simulink model "SIMULACION"  (R2025a)
settings: Solver=VariableStepAuto  StartTime=0.0  StopTime=100  RelTol=1e-3
values from neighbouring files (symbols this model uses):
  A = [0 1 0; -2.9856 -0.2654 0; -0.2985 0 0]    [Ackerman.m]    (also in L1.m = [0 1 0 0; Lab1.m = [0 1 0 0)
  Ac_poly = [0 1 0 0 ... (first row only)    [L1.m]    (also in Lab1.m)
  amp = 1    [L1.m]
  Ao_poly = [0 0 0 -den(5) ... (first row only)    [L1.m]    (also in Lab1.m)
  Ap = Ac_poly    [L1.m]    (also in Lab1.m = A)
  B = [0; 1; 0]    [Ackerman.m]    (also in L1.m = [0; 1/m; 0; -1/(m*L)]; Lab1.m = [0; 1/m; 0; -1/(m*L)])
  Bc_poly = [0; 0; 0; 1]    [L1.m]    (also in Lab1.m)
  Bo_poly = [num(5)-(den(5)*num(1)) ... (first row only)    [L1.m]    (also in Lab1.m)
  Bp = Bc_poly    [L1.m]    (also in Lab1.m = B)
  C = [1 0 0 0]    [L1.m]    (also in Lab1.m)
  Cc_poly = [num(5)-(den(5)*num(1))  num(4)-(den(4)*num(1))             num(3)-(den(3)*num(1))  num(2)-(den(2)*num(1))]    [L1.m]    (also in Lab1.m)
  Co_poly = [0 0 0 1]    [L1.m]    (also in Lab1.m)
  Cp = Cc_poly    [L1.m]    (also in Lab1.m = C)
  E = [0; M/m; 0; -M + m/L*m]    [L1.m]    (also in Lab1.m)
  sol_ki = double(sol.ki)    [L1.m]    (also in Lab1.m)
  sol_vector = double(k_valores)    [L1.m]    (also in Lab1.m)
  w = 1    [L1.m]

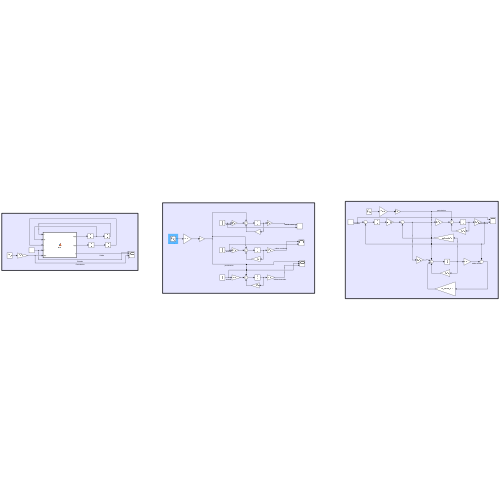
[thumbnail: Simulink's stored preview of the top-level diagram]
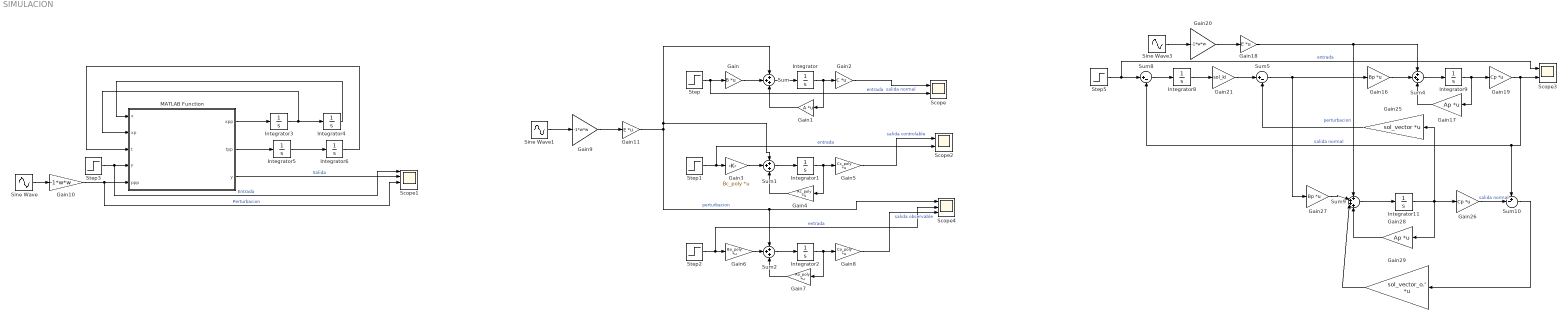
== system SIMULACION ==
  Gain : Gain  Gain=B  Multiplication=Matrix(K*u)
  Gain1 : Gain  Gain=A  Multiplication=Matrix(K*u)
  Gain10 : Gain  Gain=-1*w*w
  Gain11 : Gain  Gain=E  Multiplication=Matrix(K*u)
  Gain16 : Gain  Gain=Bp  Multiplication=Matrix(K*u)
  Gain17 : Gain  Gain=Ap  Multiplication=Matrix(K*u)
  Gain18 : Gain  Gain=E  Multiplication=Matrix(K*u)
  Gain19 : Gain  Gain=Cp  Multiplication=Matrix(K*u)
  Gain2 : Gain  Gain=C  Multiplication=Matrix(K*u)
  Gain20 : Gain  Gain=-1*w*w
  Gain21 : Gain  Gain=sol_ki
  Gain25 : Gain  Gain=sol_vector  Multiplication=Matrix(K*u)
  Gain26 : Gain  Gain=Cp  Multiplication=Matrix(K*u)
  Gain27 : Gain  Gain=Bp  Multiplication=Matrix(K*u)
  Gain28 : Gain  Gain=Ap  Multiplication=Matrix(K*u)
  Gain29 : Gain  Gain=sol_vector_o.'  Multiplication=Matrix(K*u)
  Gain3 : Gain  Gain=Bc_poly  Multiplication=Matrix(K*u)
  Gain4 : Gain  Gain=Ac_poly  Multiplication=Matrix(K*u)
  Gain5 : Gain  Gain=Cc_poly  Multiplication=Matrix(K*u)
  Gain6 : Gain  Gain=Bo_poly  Multiplication=Matrix(K*u)
  Gain7 : Gain  Gain=Ao_poly  Multiplication=Matrix(K*u)
  Gain8 : Gain  Gain=Co_poly  Multiplication=Matrix(K*u)
  Gain9 : Gain  Gain=-1*w*w
  Integrator{,1..6,8..9,11} (10 alike) : Integrator
  MATLAB Function : MATLAB Function  TreatAsAtomicUnit=on
  Scope : Scope  NumInputPorts=2
  Scope1 : Scope  NumInputPorts=4
  Scope2 : Scope  NumInputPorts=2
  Scope3 : Scope  NumInputPorts=2
  Scope4 : Scope  NumInputPorts=3
  Sine Wave : Sin  Amplitude=amp  Frequency=w  SampleTime=0
  Sine Wave1 : Sin  Amplitude=amp  Frequency=w  SampleTime=0
  Sine Wave3 : Sin  Amplitude=amp  Frequency=w  SampleTime=0
  Step{,1..3,5} (5 alike) : Step  SampleTime=0
  Sum{,1..2,4} (4 alike) : Sum  Inputs=+++
  Sum10 : Sum  Inputs=+-|
  Sum5 : Sum  Inputs=|+-
  Sum8 : Sum  Inputs=|+-
  Sum9 : Sum  Inputs=++++
  wires:
  Sum/1 -> Integrator/1
  Step/1 -> Scope/2, Gain/1  "entrada"
  Integrator/1 -> Gain1/1, Gain2/1
  Gain2/1 -> Scope/1  "salida normal"
  Gain5/1 -> Scope2/1  "salida controlable"
  Integrator1/1 -> Gain5/1, Gain4/1
  Step1/1 -> Scope2/2, Gain3/1  "entrada"
  Sum1/1 -> Integrator1/1
  Sum2/1 -> Integrator2/1
  Step2/1 -> Scope4/2, Gain6/1  "entrada"
  Integrator2/1 -> Gain7/1, Gain8/1
  Gain8/1 -> Scope4/3  "salida observable"
  MATLAB Function/1(xpp) -> Integrator3/1
  Integrator3/1 -> Integrator4/1, MATLAB Function/2(xp)
  Integrator4/1 -> MATLAB Function/1(x)
  Integrator5/1 -> Integrator6/1
  MATLAB Function/2(tpp) -> Integrator5/1
  Integrator6/1 -> MATLAB Function/3(t)
  Step3/1 -> Scope1/1, MATLAB Function/4(F)  "Entrada"
  Gain10/1 -> Scope1/3, MATLAB Function/5(ppp)  "Perturbacion"
  MATLAB Function/3(y) -> Scope1/2  "Salida"
  Sine Wave/1 -> Gain10/1
  Gain/1 -> Sum/2
  Gain3/1 -> Sum1/2
  Gain6/1 -> Sum2/2
  Gain1/1 -> Sum/3
  Gain4/1 -> Sum1/3
  Gain7/1 -> Sum2/3
  Gain11/1 -> Sum/1, Sum1/1, Scope4/1, Sum2/1  "perturbacion"
  Sine Wave1/1 -> Gain9/1
  Gain9/1 -> Gain11/1
  Gain25/1 -> Sum5/2
  Sum8/1 -> Integrator8/1
  Integrator8/1 -> Gain21/1
  Gain21/1 -> Sum5/1
  Sum5/1 -> Gain27/1, Gain16/1
  Sum4/1 -> Integrator9/1
  Step5/1 -> Scope3/1, Sum8/1  "entrada"
  Integrator9/1 -> Gain19/1, Gain17/1
  Gain19/1 -> Scope3/2, Sum10/1, Sum8/2  "salida normal"
  Gain16/1 -> Sum4/2
  Gain17/1 -> Sum4/3
  Gain18/1 -> Sum9/1, Sum4/1  "perturbacion"
  Sine Wave3/1 -> Gain20/1
  Gain20/1 -> Gain18/1
  Integrator11/1 -> Gain25/1, Gain28/1, Gain26/1
  Sum9/1 -> Integrator11/1
  Gain27/1 -> Sum9/2
  Gain28/1 -> Sum9/4
  Gain26/1 -> Sum10/2  "salida normal"
  Sum10/1 -> Gain29/1
  Gain29/1 -> Sum9/3

== matlab function SIMULACION/MATLAB Function ==
function [xpp, tpp, y] = fcn(x, xp, t, F, ppp)

k1 = 20; 
k2 = 30; 
b1 = 4; 
b2 = 3;
M = 1; 
m = 1.5; 
g = 9.81;
L = 0.3; 


xpp = (F + M*ppp+ M*g*sin(t) -(k1+k2)*x -(b1+b2)*xp)/m;

tpp = (-F - (M + m)*ppp - (M + m)*g*sin(t) + (b1 + b2)*xp + (k1 + k2)*x) / (m*L);



y = x;

end
